simulink model "TestGroup"  (R2024b)
settings: Solver=VariableStepAuto  StartTime=0.0  StopTime=45  RelTol=1e-3
undefined symbols (not defined in the file or in its folder): A_altitude, B_altitude, C_altitude, D_altitude
settings Model: Creator=hazza  LastModifiedBy=hazza

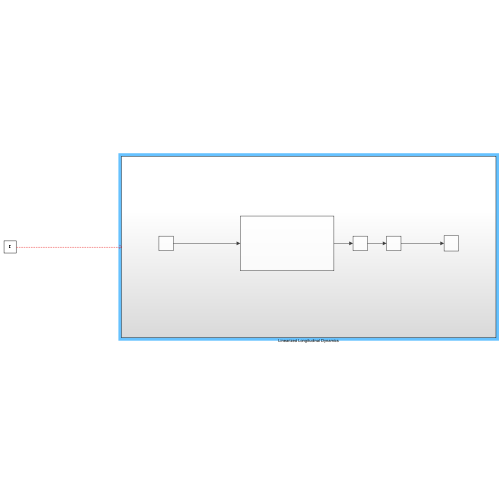
[thumbnail: Simulink's stored preview of the top-level diagram]
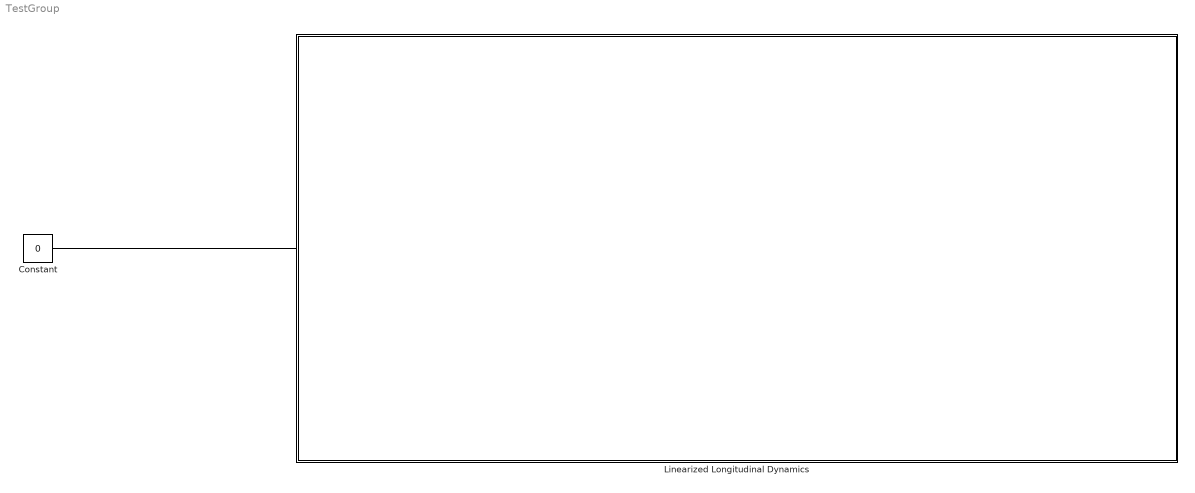
== system TestGroup ==
  Constant : Constant  Value=0
  Linearized Longitudinal Dynamics : Subsystem
  wires:
  Constant/1 -> ?

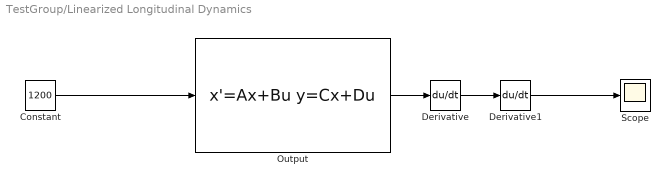
== system TestGroup/Linearized Longitudinal Dynamics ==
  Constant : Constant  Value=1200
  Derivative : Derivative
  Derivative1 : Derivative
  Output : StateSpace  A=A_altitude  B=B_altitude  C=C_altitude  D=D_altitude  InitialCondition=[1200,0,0]
  Scope : Scope
  wires:
  Constant/1 -> Output/1
  Output/1 -> Derivative/1
  Derivative/1 -> Derivative1/1
  Derivative1/1 -> Scope/1
